simulink model "Telecom2021Part2"  (R2015a)
settings: Solver=ode45  StartTime=0.0  StopTime=1000  RelTol=1e-3
settings Model: Creator=Charilaos  LastModifiedBy=Charilaos

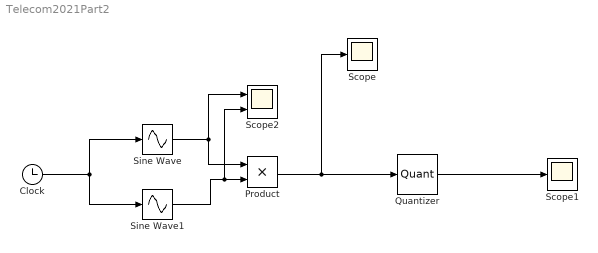
== system Telecom2021Part2 ==
  Clock : Clock
  Product : Product
  Quantizer : Quantizer  LinearizeAsGain=off
  Scope : Scope
  Scope1 : Scope
  Scope2 : Scope  NumInputPorts=2
      settings: YMin=-5~-5  YMax=5~5  SaveName=ScopeData2
  Sine Wave : Sin  TimeSource=Use external signal  Frequency=2  Phase=pi/2  SampleTime=0
  Sine Wave1 : Sin  TimeSource=Use external signal  Frequency=18  Phase=pi/2  SampleTime=0
  wires:
  Sine Wave1/1 -> Scope2/2, Product/2
  Sine Wave/1 -> Scope2/1, Product/1
  Product/1 -> Scope/1, Quantizer/1
  Quantizer/1 -> Scope1/1
  Clock/1 -> Sine Wave1/1, Sine Wave/1
